simulink model "RateAdaptiveTest"  (R2020a)
settings: Solver=FixedStepAuto  StartTime=0.0  StopTime=10.0  FixedStep=1e-3  RelTol=1e-3  EnableMultiTasking=on
settings Model: ExtModeTrigDuration=5  Creator=WinnieTrandinh  LastModifiedBy=WinnieTrandinh
settings OptimizationCC: EnhancedBackFolding=on  PassReuseOutputArgsAs=Individual arguments  ZeroExternalMemoryAtStartup=off  ZeroInternalMemoryAtStartup=off  MaxStackSize=64  OptimizeBlockOrder=speed  DifferentSizesBufferReuse=on  OptimizationCustomize=off  EfficientTunableParamExpr=on
settings DebuggingCC: ParameterTunabilityLossMsg=error
settings HardwareCC: ProdBitPerPointer=32  ProdBitPerSizeT=32  ProdBitPerPtrDiffT=32  ProdLargestAtomicInteger=Long  ProdLargestAtomicFloat=Double  ProdWordSize=32  ProdHWDeviceType=ARM Compatible->ARM Cortex
settings SFSimCC: MATLABDynamicMemAlloc=off
settings RTWCC: SystemTargetFile=ert.tlc  HardwareBoard=NXP FRDM-K64F  TemplateMakefile=ert_default_tmf  Toolchain=GNU Tools for ARM Embedded Processors
settings CodeAppCC: ForceParamTrailComments=on  IgnoreCustomStorageClasses=off  OperatorAnnotations=on  SimulinkDataObjDesc=on  SFDataObjDesc=on  InsertBlockDesc=on

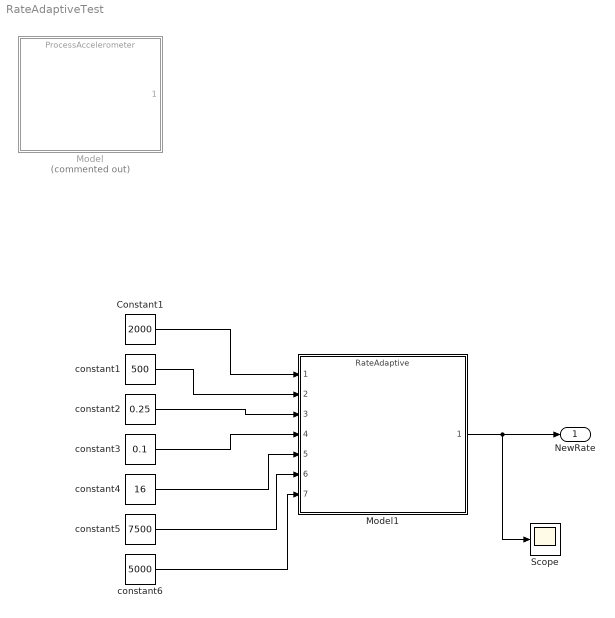
== system RateAdaptiveTest ==
  Constant1 : Constant  Value=2000
  Model : ModelReference  Commented=on  ModelNameDialog=ProcessAccelerometer.slx  SimulationMode=Normal  ModelReferenceVersion=1.6
  Model1 : ModelReference  ModelNameDialog=RateAdaptive.slx  SimulationMode=Normal  ModelReferenceVersion=1.16
  Scope : Scope
  constant1 : Constant  Value=500
  constant2 : Constant  Value=0.25
  constant3 : Constant  Value=0.1
  constant4 : Constant  Value=16
  constant5 : Constant  Value=7500
  constant6 : Constant  Value=5000
  NewRate : Outport
  wires:
  constant1/1 -> Model1/2
  constant5/1 -> Model1/6
  constant2/1 -> Model1/3
  Constant1/1 -> Model1/1
  Model1/1 -> Scope/1, NewRate/1
  constant3/1 -> Model1/4
  constant6/1 -> Model1/7
  constant4/1 -> Model1/5
